simulink library "powerlib_extras"  (Simulink 6.0)
settings: Solver=ode45  SolverMode=SingleTasking  StartTime=0.0  StopTime=10.0  RelTol=1e-3
values from neighbouring files (symbols this model uses):
  Ts = get(handles.edit1,'string')    [powergui.m]
undefined symbols (not defined in the file or in its folder): Ac, Bc, Cc, Dc, Delay_discrete, dend, DiscIntNeverNeededParam, extra_sc, j, numd, test_alpha
libraries: powerlib2 x112, powerlib_extras x70, simulink_extras x25, simulink x12, powerlib_models x8
(part 2 of 9)

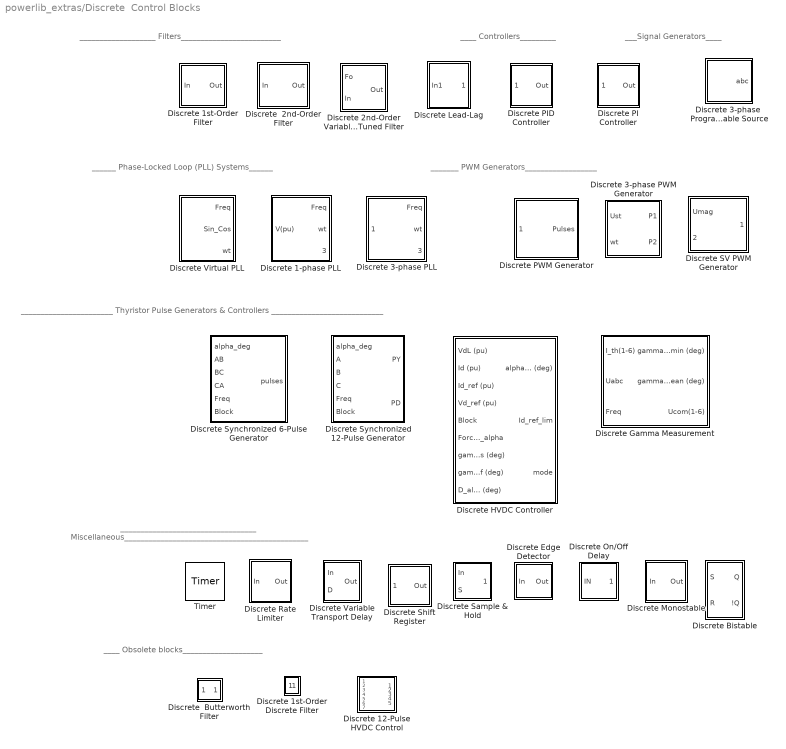
== system powerlib_extras/Discrete  Control Blocks ==
  note: ___________________ Filters_________________________
  note: ______ Phase-Locked Loop (PLL) Systems______
  note: _______________________ Thyristor Pulse Generators & Controllers ____________________________
  note: _______ PWM Generators__________________
  note: __________________________________ Miscellaneous______________________________________________
  note: ____ Controllers_________
  note: ___Signal Generators____
  note: ____ Obsolete blocks____________________
  Discrete 1-phase PLL : Subsystem  mask(Discrete 1-phase PLL){Fmin=45, Par_Init=[-45 60], ParK=[120 2800], Ts=50e-6}
      mask prompts: Fmin "Minimum frequency (Hz):"; Par_Init "Initial input:[ Phase(degrees)   Frequency(Hz) ]"; ParK "Regulator gains [ Kp  Ki ]"; Ts "Sample time:"
      mask help:
      | This Phase Locked Loop (PLL) system can be used  to synchronize on a variable frequency sinusoidal signal.
      |
      | Input 1: Normalized input signal V(pu)
      |
      | Output 1:  Measured frequency (Hz) = w/(2pi)
      | Output 2:  Ramp w.t  varying between  0 and 2*pi, synchronized on the zero-crossing (rising) of  the input signal
      | Output 3: Vector [sin(wt) cos(wt)]
      mask init:
      | Kp=ParK(1);
      | Ki=ParK(2);
      | Phase_Init=Par_Init(1);
      | Finit=Par_Init(2);
  Discrete 1st-Order Discrete Filter : Subsystem  mask(Discrete 1st-Order Filter){FilterType=Highpass, Tc=12e-3, Ts=50e-6, Initialize=off, Vac_Init=[0.8 -25 60], Vdc_Init=-0.4, PlotResponse=off, param1=[1 500 0.1]}
      mask prompts: FilterType "Filter Type:"; Tc "Time constant (s):"; Ts "Sample time:"; Initialize "Initialize filter states"; Vac_Init "AC initial input: [ Mag  Phase(degrees)  Freq(Hz) ]"; Vdc_Init "DC Initial input:"; PlotResponse "Plot filter response"; param1 "Frequency range(Hz) : [Start  End  Inc.]"
      mask init:
      | switch FilterType
      | case 1, % Lowpass
      |     X=[0 1 2 3 4];
      |     Y=[-2 -2 -3 -4 -4];
      |     numc=1;
      |     denc=[Tc 1];
      | case 2,   % Highpass
      |     X=[0 1 2 3 4];
      |     Y=[-4 -4 -3 -2 -2];
      |     numc=[1 0];
      |     denc=[1 1/Tc];
      | end
      | %
      | [Ac,Bc,Cc,Dc]=tf2ss(numc,denc);
      | %
      | %  Conversion to discrete transfer function
      | nstates = size(Ac,1);
      | invexp = inv(eye(nstates) - (Ts/2)*Ac);
      | Ad = invexp*(eye(nstates) + (Ts/2)*Ac);
      | Bd = invexp*Bc;
      | Cd = Cc*invexp*Ts;
      | Dd = Cc*invexp*Bc*(Ts/2) + Dc;
      | %
      | if Initialize==1  % Compute initial conditions on states
      |     u1=Vac_Init(1)*exp(j*Vac_Init(2)*pi/180);
      |     u2=Vdc_Init*exp(j*90*pi/180);
      |     u=u1+u2;
      |     u0=imag(u); % input at  t=0;
      |     I=eye(size(Ac));
      |     sI1=I*j*(2*pi*Vac_Init(3));
      |     sI2=I*j*0;
      |     x=inv(sI1-Ac)*Bc*u1 + inv(sI2-Ac)*Bc*u2;
      |     x0c=imag(x);
      |     x0d=(I-Ac*Ts/2)*x0c/Ts - Bc/2*u0;
      | else
      |     x0d=0;
      | end
      | 
      | %
      | if PlotResponse==1 % Plot frequency and step response
      | t=[0:Tc/1000:7*Tc];
      | f=param1(1):param1(3):param1(2);
      | w=2*pi*f;
      | switch FilterType
      | 	case 1, % Lowpass
      | 		Ystep=1 - exp(-t/Tc);
      | 		RepFreq=1./(1+Tc*j.*w);
      | 	case 2,   % Highpass
      | 		Ystep=exp(-t/Tc);
      | 		RepFreq=1./(1 + (1./(Tc*j.*w)));
      | end
      | %
      | Mag=abs(RepFreq);
      | Pha=angle(RepFreq)*180/pi;
      | %
      | figure(1)
      | subplot(2,1,1)
      | plot(f,Mag)
      | grid
      | title('Bode Diagram')
      | ylabel('Magnitude')
      | subplot(2,1,2)
      | plot(f,Pha)
      | ylabel('Phase (deg)')
      | xlabel('Frequency (Hz)')
      | grid
      | figure(2)
      | plot(t,Ystep)
      | grid
      | ylabel('Amplitude')
      | xlabel('Time (s)')
      | title('Step Response')
      | end
      mask StyleString: popup(Lowpass|Highpass),edit,edit,checkbox,edit,edit,checkbox,edit
      mask CallbackString: |||p4=get_param(gcb,'Initialize');if strcmp(p4,'on');visible={'on','on','on','on','on','on','on',get_param(gcb,'PlotResponse')};else;visible={'on','on','on','on','off','off','on',get_param(gcb,'PlotResponse')};end;set_param(gcb,'MaskVisibilities',visible)|||p7=get_param(gcb,'PlotResponse');if strcmp(p7,'on');visible={'on','on','on','on',get_param(gcb,'Initialize'),get_param(gcb,'Initialize'),'on','on'};else;visible={'on','on','on','on',get_param(gcb,'Initialize'),get_param(gcb,'Initialize'),'on','off'};end;set_param(gcb,'MaskVisibilities',visible)|
      mask Display: plot(X,Y);
  Discrete 1st-Order Filter : Subsystem  mask(Discrete 1st-Order Filter){FilterType=Highpass, Tc=12e-3, Ts=50e-6, Initialize=off, Vac_Init=[0.8 -25 60], Vdc_Init=-0.4, PlotResponse=off, param1=[1 500 0.1]}
      mask prompts: FilterType "Filter Type:"; Tc "Time constant (s):"; Ts "Sample time:"; Initialize "Initialize filter states"; Vac_Init "AC initial input: [ Mag  Phase(degrees)  Freq(Hz) ]"; Vdc_Init "DC Initial input:"; PlotResponse "Plot filter response"; param1 "Frequency range(Hz) : [Start  End  Inc.]"
      mask init: same as powerlib_extras/Discrete  Control Blocks/Discrete 1st-Order Discrete Filter
      mask StyleString: popup(Lowpass|Highpass),edit,edit,checkbox,edit,edit,checkbox,edit
      mask CallbackString: |||p4=get_param(gcb,'Initialize');if strcmp(p4,'on');visible={'on','on','on','on','on','on','on',get_param(gcb,'PlotResponse')};else;visible={'on','on','on','on','off','off','on',get_param(gcb,'PlotResponse')};end;set_param(gcb,'MaskVisibilities',visible)|||p7=get_param(gcb,'PlotResponse');if strcmp(p7,'on');visible={'on','on','on','on',get_param(gcb,'Initialize'),get_param(gcb,'Initialize'),'on','on'};else;visible={'on','on','on','on',get_param(gcb,'Initialize'),get_param(gcb,'Initialize'),'on','off'};end;set_param(gcb,'MaskVisibilities',visible)|
      mask Display: plot(X,Y);
  Discrete 2nd-Order Variable-Tuned Filter : Subsystem  mask(Discrete 2nd-Order Variable-Tuned Filter){FilterType=Bandpass, Fo=60, Zeta=1, Ts=50e-6, Initialize=off, Par_Init=[1.2 -30 30], Vdc=0}
      mask prompts: FilterType "Type of filter:"; Fo "Initial cut-off frequency Fo (Hz):"; Zeta "Damping factor Zeta ( Q = 1 / (2*Zeta) ):"; Ts "Sample Time: (s)"; Initialize "Initialize filter states"; Par_Init "AC initial input: [ Mag  Phase(degrees)  Freq(Hz) ]"; Vdc "DC initial input:"
      mask init:
      | switch FilterType
      | case 1, % Lowpass
      |        X=[0 1 2 3 4];
      |        Y=[-2 -2 -3 -4 -4];
      |  case 2,   % Highpass
      |        X=[0 1 2 3 4];
      |        Y=[-4 -4 -3 -2 -2];
      |     case 3,   % Bandpass
      |        X=[0 1 2 3 4 5 ];
      |        Y=[-3 -3 -2 -2 -3 -3];
      |     case 4,  %Bandstop (Notch)
      |        X=[0 1 2 3 4 5 ];
      |        Y=[-2 -2 -3 -3 -2 -2];
      |  end
      | Correction=3.549e6*Ts*Ts/60/60/60;
      | if Initialize==1
      | Vin=Par_Init(1)*(cos(Par_Init(2)*pi/180) + j*sin(Par_Init(2)*pi/180));
      | I=Vin/2/Zeta/(2*pi*Par_Init(3));
      | Wo=2*pi*Fo;
      | W=2*pi*Par_Init(3);
      | R=2*Zeta*Wo;
      | L=1;
      | C=1/(Wo*Wo);
      | I=Vin/(R + j*W*L -j/C/W);
      | Iinit=imag(I);
      | VL=imag(I * j*W*L);
      | VC=imag(I * -j/W/C)+ Vdc;
      | else
      | VC=0;
      | VL=0;
      | Iinit=0;
      | end
      mask StyleString: popup(Lowpass|Highpass|Bandpass|Bandstop (Notch)),edit,edit,edit,checkbox,edit,edit
      mask CallbackString: ||||p5=get_param(gcb,'Initialize');if strcmp(p5,'on');visible={'on','on','on','on','on','on','on'};else;visible={'on','on','on','on','on','off','off'};end;set_param(gcb,'MaskVisibilities',visible)||
      mask Display: plot(X,Y);
  Discrete 3-phase  Programmable Source : Subsystem  mask(Discrete 3-phase Programmable Source){Par_Vps=[1.0 -20  60], VariationEntity=Amplitude, VariationType=Step, VariationStep=-0.5, VariationRate=10, VariationMag=0.3, VariationFreq=2, Par_Timing_Variation=[0.1 1.2], SinglePhase=on, Yampli=[1 0.2 1.2 1.0], Xtime=[0 0.1 0.15 0.2], HarmonicGeneration=off, Par_HarmoA=[3 0.2 -25 0], Par_HarmoB=[2 0.15 35 2], Par_Timing_Harmo=[0.05  3], Ts=50e-6}
      mask prompts: Par_Vps "Positive-sequence: [ Amplitude  Phase(degrees)   Freq. (Hz) ]"; VariationEntity "Time variation of:"; VariationType "Type of variation:"; VariationStep "Step magnitude:"; VariationRate "Rate of change (value/s):"; VariationMag "Amplitude of the modulation:"; VariationFreq "Frequency of the modulation(Hz):"; Par_Timing_Variation "Variation timing (s) : [ Start   End ]"; SinglePhase "1-phase only"; Yampli "Amplitude values:"; Xtime "Time values:"; HarmonicGeneration "Harmonic generation:"; Par_HarmoA "A:  [ Order(n)   Amplitude  Phase(degrees)  Seq(0, 1 or 2) ]"; Par_HarmoB "B:  [ Order(n)   Amplitude  Phase(degrees)  Seq(0, 1 or 2) ]"; Par_Timing_Harmo "Harmonic timing (s) : [ Start   End ]"; Ts "Sample time:"
      mask help: Use this discrete block to generate a set of three-phase sinusoidal voltages or currents a, b and c. Time variation for the amplitude, phase and frequency of the fundamental can be pre-programmed. In addition, two harmonics can be surimposed on the fundamental.
      mask init:
      | Mag_Vps=Par_Vps(1);
      | Phase_Vps=Par_Vps(2);
      | Freq_Vps=Par_Vps(3);
      | 
      | Ton_Variation=Par_Timing_Variation(1);
      | Toff_Variation=Par_Timing_Variation(2);
      | n_HarmoA=Par_HarmoA(1);
      | Mag_HarmoA=Par_HarmoA(2);
      | Phase_HarmoA=Par_HarmoA(3);
      | Seq_HarmoA=Par_HarmoA(4);
      | if n_HarmoA==0
      |     Phase_HarmoA=90;
      |     Seq_HarmoA=0;
      | end
      | n_HarmoB=Par_HarmoB(1);
      | Mag_HarmoB=Par_HarmoB(2);
      | Phase_HarmoB=Par_HarmoB(3);
      | Seq_HarmoB=Par_HarmoB(4);
      | if n_HarmoB==0
      |     Phase_HarmoB=90;
      |     Seq_HarmoB=0;
      | end
      | Ton_Harmo=Par_Timing_Harmo(1);
      | Toff_Harmo=Par_Timing_Harmo(2);
      | 
      | if Xtime(1)~=0,
      | Xtime=[0 Xtime];
      | Yampli=[0 Yampli];
      | end
      | n=length(Xtime); vec_dt= [Xtime,0] - [0,Xtime] ; vec_dt=vec_dt(2:n);
      mask StyleString: edit,popup(None|Amplitude|Phase|Frequency),popup(Step|Ramp|Modulation|Table of time-amplitude pairs),edit,edit,edit,edit,edit,checkbox,edit,edit,checkbox,edit,edit,edit,edit
      mask CallbackString: |parametres=get_param(gcb,'MaskValues');p2=parametres{2};p3=parametres{3};p12=parametres{12};if strcmp(p3,'Step');param4='on';param5='off';param6='off';param7='off';param8='on';param9='off';param10='off';param11='off';elseif strcmp(p3,'Ramp');param4='off';param5='on';param6='off';param7='off';param8='on';param9='off';param10='off';param11='off';elseif strcmp(p3,'Modulation');param4='off';param5='off';param6='on';param7='on';param8='on';param9='off';param10='off';param11='off';else;param4='off';param5='off';param6='off';param7='off';param8='off';param9='on';param10='on';param11='on';end;if strcmp(p2,'None');param3='off';param4='off';param5='off';param6='off';param7='off';param8='off';param9='off';param10='off';param11='off';else;param3='on';end;if strcmp(p12,'on');param13='on';param14='on';param15='on';else;param13='off';param14='off';param15='off';end;visible={'on','on',param3,param4,param5,param6,param7,param8,param9,param10,param11,'on',param13,param14,param15,'on'};set_param(gcb,'MaskVisibilities',visible)|parametres=get_param(gcb,'MaskValues');p2=parametres{2};p3=parametres{3};p12=parametres{12};if strcmp(p3,'Step');param4='on';param5='off';param6='off';param7='off';param8='on';param9='off';param10='off';param11='off';elseif strcmp(p3,'Ramp');param4='off';param5='on';param6='off';param7='off';param8='on';param9='off';param10='off';param11='off';elseif strcmp(p3,'Modulation');param4='off';param5='off';param6='on';param7='on';param8='on';param9='off';param10='off';param11='off';else;param4='off';param5='off';param6='off';param7='off';param8='off';param9='on';param10='on';param11='on';end;if strcmp(p2,'None');param3='off';param4='off';param5='off';param6='off';param7='off';param8='off';param9='off';param10='off';param11='off';else;param3='on';end;if strcmp(p12,'on');param13='on';param14='on';param15='on';else;param13='off';param14='off';param15='off';end;visible={'on','on',param3,param4,param5,param6,param7,param8,param9,param10,param11,'on',param13,param14,param15,'on'};set_param(gcb,'MaskVisibilities',visible)|||||||||parametres=get_param(gcb,'MaskValues');p2=parametres{2};p3=parametres{3};p12=parametres{12};if strcmp(p3,'Step');param4='on';param5='off';param6='off';param7='off';param8='on';param9='off';param10='off';param11='off';elseif strcmp(p3,'Ramp');param4='off';param5='on';param6='off';param7='off';param8='on';param9='off';param10='off';param11='off';elseif strcmp(p3,'Modulation');param4='off';param5='off';param6='on';param7='on';param8='on';param9='off';param10='off';param11='off';else;param4='off';param5='off';param6='off';param7='off';param8='off';param9='on';param10='on';param11='on';end;if strcmp(p2,'None');param3='off';param4='off';param5='off';param6='off';param7='off';param8='off';param9='off';param10='off';param11='off';else;param3='on';end;if strcmp(p12,'on');param13='on';param14='on';param15='on';else;param13='off';param14='off';param15='off';end;visible={'on','on',param3,param4,param5,param6,param7,param8,param9,param10,param11,'on',param13,param14,param15,'on'};set_param(gcb,'MaskVisibilities',visible)||||
  Discrete 3-phase PLL : Subsystem  mask(Discrete 3-phase PLL){Fmin=45, Par_Init=[-45 60], ParK=[60 1400], Ts=50e-6}
      mask prompts: Fmin "Minimum frequency (Hz):"; Par_Init "Initial inputs:[ Phase(degrees)   Frequency(Hz) ]"; ParK "Regulator gains [ Kp  Ki ]"; Ts "Sample time:"
      mask help:
      | This Phase Locked Loop (PLL) system can be used  to synchronize on a set of variable frequency, three-phase sinusoidal signals.
      |
      | Input 1: Vector containing the normalized
      |              three-phase signals [Va Vb Vc]
      | Output 1:  Measured frequency (Hz) = w/(2pi)
      | Output 2:  Ramp w.t   varying between  0 and 2*pi,
      | synchronized on zero crossings of the fundamental (positive-sequence) of phase A.
      | Output 3: Vector [sin(wt) cos(wt)]
      mask init:
      | Kp=ParK(1);
      | Ki=ParK(2);
      | Phase_Init=Par_Init(1);
      | Finit=Par_Init(2);
  Discrete Bistable : Subsystem  AncestorBlock=my_linear/BETA/Flip flop [R]  mask(Discrete Bistable Flip-Flop (Priority to Set or Reset)){priority=Set, ic=0, Ts=50e-6}
      mask prompts: priority "Priority to input:"; ic "Initial Q output (0/1):"; Ts "Sample time:"
      mask help:
      | SR Flip-Flop block, with priority given either  to the Set  (S) or Reset  (R) input.
      |
      | Priority to Set: If inputs S (set) and R (reset) are TRUE (1) simultaneously, the output Q is set to TRUE (1).
      |
      | Priority to Reset: If inputs S (set) and R (reset) are TRUE (1) simultaneously, the output Q is reset to FALSE (0).
      |
      | The  Q! output  is the complement of the Q output.
      | The initial value of the Q output  is specified by the parameter "Initial Q output".
      mask init:
      | if (priority==1)   % RESET
      |  str1 = '[R]';
      |  str2 = 'S';
      | else
      | str1= 'R';
      | str2 = '[S]';
      | end
      mask StyleString: popup(Reset|Set),edit,edit
      mask Display:
      | plot(0,0,100,100);
      | text(5,25,str1);
      | text(5,75,str2);
      | text(72,25,'!Q');
      | text(78,75,'Q');
  Discrete Edge Detector : Subsystem  mask(Discrete Edge Detector){model=Rising, ic=0, Ts=50e-6}
      mask prompts: model "Edge:"; ic "Input at t = -Ts:"; Ts "Sample time Ts:"
      mask help:
      | This block compares its present input to its previous input.
      |
      | If the input  is a logic signal (TRUE (1) or FALSE (0), the output is a one-step boolean signal TRUE  when  the specified edge (Rising, Falling or Either)  is detected.
      |
      | This block can also be used to detect the slope polarity of a continuous signal. For example, if the specified edge is  "Rising", the output is TRUE as long as the slope of the input signal is positive.
      |
      | The input value at time step preceeding t=0 is specified by the parameter "Input at t=-Ts"
      mask init: same as powerlib_extras/Control  Blocks/Edge Detector
      mask StyleString: popup(Rising|Falling|Either),edit,edit
      mask Display: plot(0,0,100,100, X1,Y1,X2,Y2,X3,Y3,X4,Y4);
  Discrete Lead-Lag : Subsystem  mask(Discrete Lead-Lag Controller){T1=5e-3, T2=20e-3, V_Init=0, Ts=50e-6}
      mask prompts: T1 "Time constant T1 (s):"; T2 "Time constant T2 (s):"; V_Init "Initial input and output:"; Ts "Sample time (s):"
      mask help:
      | This block implements a discrete lead-lag controller:
      |
      |          1+T1s
      | H(s)= ------
      |          1+T2s
      |
      | States are initialized according to initial input anf output value so that simulation starts in steady state.
      mask init:
      | numc=[T1 1];
      | denc=[T2 1];
      | [Ac,Bc,Cc,Dc]=tf2ss(numc,denc);
      | 
      | %  Conversion to discrete transfer function
      | nstates = size(Ac,1);
      | invexp = inv(eye(nstates) - (Ts/2)*Ac);
      | Ad = invexp*(eye(nstates) + (Ts/2)*Ac);
      | Bd = invexp*Bc;
      | Cd = Cc*invexp*Ts;
      | Dd = Cc*invexp*Bc*(Ts/2) + Dc;
      | %
      | % Compute Initial states
      | I=eye(size(Ac));
      | x0c=inv(-Ac)*Bc*V_Init;
      | x0d=(I-Ac*Ts/2)*x0c/Ts - Bc/2*V_Init;
      | 
      | if T1==0 & T2==0, Dd=1; end
      mask Display: disp('1+T1s\n---\n1+T2s')
  Discrete Monostable : Subsystem  mask(Discrete Monostable Flip-Flop){EdgeDetect=Rising, t_mono=0.015, ic=0, Ts=50e-6}
      mask prompts: EdgeDetect "Edge detection"; t_mono "Pulse duration (s):"; ic "Input at t = -Ts:"; Ts "Sample time Ts:"
      mask help:
      | After being triggered  by the specified edge (Rising, Falling or Either), this block outputs a pulse (TRUE signal) for the time specified by parameter "Pulse duration".
      | If the specified edge is detected while the output is TRUE, the monostable is not retriggered
      |
      | The input value (0/1) at time step preceeding t = 0 is specified by the parameter "input at t = -Ts.
      mask init: same as powerlib_extras/Control  Blocks/Monostable
      mask StyleString: popup(Rising|Falling|Either),edit,edit,edit
      mask Display:
      | plot(0,0,100,100,[100 75 75 25 25 0],[25 25 50 50 25 25]-0,X1,Y1,X2,Y2,X3,Y3,X4,Y4);
      | text(45,37,'T');
      | text(15,15,str);
  Discrete On/Off Delay : Subsystem  AncestorBlock=extra_sc/Delay_discrete  mask(Discrete On/Off Delay ){type_delay=On delay, delay=0.01, ic=0, Ts=50e-6}
      mask prompts: type_delay "Type:"; delay "Time delay:"; ic "Input at t = -Ts (0/1):"; Ts "Sample time Ts:"
      mask help:
      | Apply a delay on the input signal when the input changes to TRUE (1) or FALSE (0).
      |
      | On delay: When the input becomes TRUE, the output becomes TRUE after the specified time delay as long as the input is still TRUE. If the input becomes FALSE before the time delay has expired , the output stays FALSE.
      |
      | Off delay: When the input becomes FALSE, the output becomes FALSE after the specified time delay as long as the input is still FALSE. If the input becomes TRUE before the time delay has expired , the output stays TRUE.
      |
      | The input value (0/1) at time step preceeding t=0 is specified by the parameter "input at t = -Ts".
      mask init:
      | str=sprintf('%g %c',delay,'s');
      mask StyleString: popup(On delay|Off delay),edit,edit,edit
      mask Display:
      | plot(0,0,100,100,[10,10,10,90,90,90],[60,40,50,50,40,60]);
      | text(25+(type_delay-1)*50,80,'t');
      | text(15,20,str);
  Discrete PI Controller : Subsystem  mask(Discrete PI Controller){Kp=0.1, Ki=1, Par_Limits=[1e6 -1e6], Init=0, Ts=50e-6}
      mask prompts: Kp "Proportional gain (Kp):"; Ki "Integral gain (Ki):"; Par_Limits "Output limits: [ Upper   Lower ]"; Init "Output initial value:"; Ts "Sample time:"
      mask help: This block implements a discrete PI controller.
      mask init:
      | UpperLimit=Par_Limits(1);
      | LowerLimit=Par_Limits(2);
      mask Display: disp('PI');
  Discrete PID Controller : Subsystem  mask(Discrete PID Controller){Kp=0.1, Ki=1, Kd=0, TcD=0.5e-3, Par_Limits=[1e6 -1e6], Init=0, Ts=50e-6}
      mask prompts: Kp "Proportional gain (Kp):"; Ki "Integral gain (Ki):"; Kd "Derivative gain (Kd):"; TcD "Time constant for derivative (s):"; Par_Limits "Output limits: [ Upper   Lower ]"; Init "Output initial value:"; Ts "Sample time:"
      mask help: This block implements a discrete PID controller.
      mask init:
      | UpperLimit=Par_Limits(1);
      | LowerLimit=Par_Limits(2);
      mask Display: disp('PID');
  Discrete PWM Generator : Subsystem  mask(Discrete PWM Generator){GeneratorMode=2-arm  bridge (4 pulses), Fc=1080, Ts=5e-6, Internal=off, mIndex=0.4, Freq=60, Phase=0}
      mask prompts: GeneratorMode "Generator Mode"; Fc "Carrier frequency (Hz):"; Ts "Sample time:"; Internal "Internal generation of modulating signal(s)"; mIndex "Modulation index  (0<m<1) :"; Freq "Frequency of output voltage (Hz)"; Phase "Phase of output voltage (degrees)"
      mask help:
      | This discrete block generates pulses for carrier-based PWM (Pulse Width Modulation), self-commutated IGBTs,GTOs or FETs bridges.
      |
      | Depending on the number of bridge arms selected in the "Generator Mode" parameter, the block can be used either for single-phase or three-phase PWM control.
      |
      | Press Help for details on input(s) and outputs.
      |
      | See psb1phPWM and psb3phPWM demos respectively  for application examples of single-phase and three-phase inverters using this block.
      mask init:
      | powericon('psbcbtransfo',gcb,'Discrete PWM Generator')
      | if Freq==0
      |     Phase=90;
      | end
      | switch GeneratorMode
      | case 1,
      |     Internal_Phase=0;
      |    Signal_PortWidth=1;
      |    Select1_Elements=[1 2];
      |    Select1_PortWidth=2;
      |    Select3_Elements=[1 2];
      |    Select3_PortWidth=4;
      | case 2,
      |     Internal_Phase=0;
      |     Signal_PortWidth=1;
      |     Select1_Elements=[1 2];
      |     Select1_PortWidth=2;
      |     Select3_Elements=[1 2 3 4];
      |     Select3_PortWidth=4;
      | case 3,
      |     Internal_Phase=[0 -2*pi/3 2*pi/3];
      |     Signal_PortWidth=3;
      |     Select1_Elements=[1 4 2 5 3 6];
      |     Select1_PortWidth=6;
      |    Select3_Elements=[1 2 3 4 5 6];
      |    Select3_PortWidth=12;
      | case 4,
      |     Internal_Phase=[0 -2*pi/3 2*pi/3];
      |     Signal_PortWidth=3;
      |     Select1_Elements=[1 4 2 5 3 6];
      |     Select1_PortWidth=6;
      |    Select3_Elements=[1 2 3 4 5 6 7 8 9 10 11 12];
      |    Select3_PortWidth=12;
      | end
      mask Help:
      | The output pulses are a vector (with values=0 or 1). Depending on the selected "Generator Mode", the output vector contains:
      | For a 1-arm  bridge: Two pulses. Pulse 1 is for the upper switch and pulse 2 is for the lower switch.
      | For a 2-arm  bridge: Four pulses. Pulses 1 and 3 are respectively for the upper switches of the first and second arm. Pulses 2 and 4 are for the lower switches.
      | For a 3-arm  bridge: Six pulses. Pulses 1,3 and 5 are respectively for the upper switches of the first,second and third arm. Pulses 2,4 and 6 are for the lower switches.
      | For double 3-arm bridges: Twelve pulses.The first six pulses (pulses 1 to 6) must be sent to the first 3-arm bridge and the last six (pulses 7 to 12) to the second 3-arm bridge.
      | 
      | By selecting "Internal generation" you can can control the modulation index m, frequency and phase of the output voltage  from the internal parameters (m, Freq and Phase). Otherwise, external signals are used for pulse generation. The width of the input vector must be 1 for single phase bridges ( 1-arm or 2-arm)  and 3 for 3-phase bridges  (single or double bridge).
      mask StyleString: popup(1-arm  bridge (2 pulses)|2-arm  bridge (4 pulses)|3-arm  bridge (6 pulses)|Double 3-arm  bridges (12 pulses)),edit,edit,checkbox,edit,edit,edit
      mask CallbackString: |||powericon('psbcbtransfo',gcb,'Discrete PWM Generator',[])|||
  Discrete Rate Limiter : Subsystem  mask{R=2000, F=-2000, Vinit=0, Ts=50e-6}
      mask prompts: R "Rising slew rate:"; F "Falling slew rate:"; Vinit "Initial input:"; Ts "Sample time:"
      mask help: DISCRETE BLOCK : Limit rising and falling rates of signal
      mask init:
      | UpperLimit=R*Ts;
      | LowerLimit=F*Ts;
      mask Display: disp('Discrete\nRate\nLimiter')
  Discrete Sample & Hold : Subsystem  mask(Discrete Sample & Hold ){ic=0, Ts=50e-6}
      mask prompts: ic "Initial condition:"; Ts "Sample time:"
      mask help: The output follows input 1 (In) as long as input 2 (S) is TRUE (1) . The output is held when input 2 becomes FALSE (0). The output initial value is specified by the parameter "Initial condition".
      mask Display: disp('S/H')
  Discrete Shift Register : Subsystem  mask(Discrete Shift Register){NSamples=32, InitialValue=0, Ts=50e-6}
      mask prompts: NSamples "Number of samples N :"; InitialValue "Initial inputs:"; Ts "Sample time Ts:"
      mask help:
      | This block implements a discrete shift register (Serial input/ Parallel output). The block accepts a vectorized input of Nsig signals.
      |
      | The block output is a vector (dimension N*Nsig) containing the last N samples of the Nsig input signals in the following order
      | [u1(k), u1(k-1), ..., u1(k-(N-1)),  u2(k), u2(k-1), ...]
      |
      | The (N-1) samples preceding time zero are set to the  value specified in the "Initial inputs" parameter.
  Discrete Virtual PLL : Subsystem  mask(Discrete Virtual PLL){Freq=60, Phase=30, Ts=50e-6}
      mask prompts: Freq "Frequency (Hz):"; Phase "Phase (degrees):"; Ts "Sample time:"
      mask help:
      | This virtual PLL has no input signal. The block simulates the outputs of an actual PLL by  using the parameters specified in the mask.
      |
      | Output 1: Frequency (Hz)
      | Output 2: Vectorized output  [sin(wt)  cos(wt)]
      | Output 3: wt in rad/s (varying from 0 to 2*pi)
  Discrete  2nd-Order Filter : Subsystem  mask(Discrete 2nd-Order Filter){FilterType=Lowpass, Fo=200, Zeta=0.707, Ts=50e-6, Initialize=off, Vac_Init=[0.8 -25 60], Vdc_Init=-0.4, PlotResponse=off, param1=[1 500 1]}
      mask prompts: FilterType "Filter Type:"; Fo "Cut-off frequency (Hz):"; Zeta "Damping factor Zeta ( Q = 1 / (2*Zeta) ):"; Ts "Sample time:"; Initialize "Initialize filter states"; Vac_Init "AC initial input: [ Mag  Phase(degrees)  Freq(Hz) ]"; Vdc_Init "DC Initial input:"; PlotResponse "Plot filter response"; param1 "Frequency range(Hz) : [Start  End  Inc.]"
      mask init:
      | str=sprintf(' Fo=%iHz\n\n',Fo);
      | Wo=2*pi*Fo;
      | switch FilterType
      | case 1, % Lowpass
      |        X=[0 1 2 3 4];
      |        Y=[-2 -2 -3 -4 -4];
      |        n2=0;n1=0;n0=Wo*Wo;
      |        d2=1;d1=2*Zeta*Wo;d0=Wo*Wo;
      | 	   Ystep=1;
      |  case 2,   % Highpass
      |        X=[0 1 2 3 4];
      |        Y=[-4 -4 -3 -2 -2];
      |        n2=1;n1=0;n0=0;
      |        d2=1;d1=2*Zeta*Wo;d0=Wo*Wo;
      | 	   Ystep=2;
      |     case 3,   % Bandpass
      |        X=[0 1 2 3 4 5 ];
      |        Y=[-3 -3 -2 -2 -3 -3];
      |        n2=0;n1=2*Zeta*Wo;n0=0;
      |        d2=1;d1=2*Zeta*Wo;d0=Wo*Wo;
      | 	   Ystep=3;
      |     case 4,  %Bandstop (Notch)
      |        X=[0 1 2 3 4 5 ];
      |        Y=[-2 -2 -3 -3 -2 -2];
      |        n2=1;n1=0;n0=Wo*Wo;
      |        d2=1;d1=2*Zeta*Wo;d0=Wo*Wo;
      | 	   Ystep=4;
      |     end
      | %
      | numc=[n2 n1 n0];
      | denc=[d2 d1 d0];
      | [Ac,Bc,Cc,Dc]=tf2ss(numc,denc);
      | %
      | %  Conversion to discrete transfer function
      | nstates = size(Ac,1);
      | invexp = inv(eye(nstates) - (Ts/2)*Ac);
      | Ad = invexp*(eye(nstates) + (Ts/2)*Ac);
      | Bd = invexp*Bc;
      | Cd = Cc*invexp*Ts;
      | Dd = Cc*invexp*Bc*(Ts/2) + Dc;
      | %
      | if Initialize==1  % Compute initial conditions on states
      | u1=Vac_Init(1)*exp(j*Vac_Init(2)*pi/180);
      | u2=Vdc_Init*exp(j*90*pi/180);
      | u=u1+u2;
      | u0=imag(u); % input at  t=0;
      | I=eye(size(Ac));
      | sI1=I*j*(2*pi*Vac_Init(3));
      | sI2=I*j*0;
      | x=inv(sI1-Ac)*Bc*u1 + inv(sI2-Ac)*Bc*u2;
      | x0c=imag(x);
      | x0d=(I-Ac*Ts/2)*x0c/Ts - Bc/2*u0;
      | else
      | x0d=0;
      | end
      | %
      | if PlotResponse==1 % Plot frequency and step response
      | if Zeta==1
      | 	z=1+1e-12;
      | else
      | 	z=Zeta;
      | end
      | wn=Wo;
      | t=[0:1/(z*wn)/1000:7/(z*wn)];
      | f=param1(1):param1(3):param1(2);
      | w=2*pi*f;
      | switch FilterType
      | 	case 1, % Lowpass
      | 		Ystep=wn^2*(1/wn^2+1/(4*z^2*wn^2-4*wn^2)^(1/2)*(1/(-z*wn+1/2*(4*z^2*wn^2-4*wn^2)^(1/2))*exp((-z*wn+1/2*(4*z^2*wn^2-4*wn^2)^(1/2))*t)-1/(-z*wn-1/2*(4*z^2*wn^2-4*wn^2)^(1/2))*exp((-z*wn-1/2*(4*z^2*wn^2-4*wn^2)^(1/2))*t)));
      | 		numFreq=wn^2;
      | 	case 2,   % Highpass
      | 		Ystep=-exp(-z*wn*t)/(z-1)/(z+1).*cos((-wn^2*(z-1)*(z+1))^(1/2)*t)+exp(-z*wn*t)/(z-1)/(z+1)*z^2.*cos((-wn^2*(z-1)*(z+1))^(1/2)*t)+z/wn*exp(-z*wn*t)/(z-1)/(z+1)*(wn^2-z^2*wn^2)^(1/2).*sin((-wn^2*(z-1)*(z+1))^(1/2)*t);
      | 		numFreq=-w.^2;
      | 	case 3,   % Bandpass
      | 		Ystep=2*z*wn/(4*z^2*wn^2-4*wn^2)^(1/2)*(exp((-z*wn+1/2*(4*z^2*wn^2-4*wn^2)^(1/2))*t)-exp((-z*wn-1/2*(4*z^2*wn^2-4*wn^2)^(1/2))*t));
      | 		numFreq=2*Zeta*wn.*w*j;
      | 	case 4,  %Bandstop (Notch)
      | 		Ystep=1+2*z/wn*exp(-z*wn*t)/(z-1)/(z+1)*(wn^2-z^2*wn^2)^(1/2).*sin((-wn^2*(z-1)*(z+1))^(1/2)*t);	
      | 		numFreq=wn^2-w.^2;
      | end
      | %
      | denFreq=(wn^2-w.^2) + 2*Zeta*wn*j.*w;
      | RepFreq=numFreq./denFreq;
      | Mag=abs(RepFreq);
      | Pha=angle(RepFreq)*180/pi;
      | %
      | figure(1)
      | subplot(2,1,1)
      | plot(f,Mag)
      | grid
      | title('Bode Diagram')
      | ylabel('Magnitude')
      | subplot(2,1,2)
      | plot(f,Pha)
      | ylabel('Phase (deg)')
      | xlabel('Frequency (Hz)')
      | grid
      | figure(2)
      | plot(t,real(Ystep))
      | grid
      | ylabel('Amplitude')
      | xlabel('Time (s)')
      | title('Step Response')
      | end
      mask StyleString: popup(Lowpass|Highpass|Bandpass|Bandstop (Notch)),edit,edit,edit,checkbox,edit,edit,checkbox,edit
      mask CallbackString: ||||p5=get_param(gcb,'Initialize');if strcmp(p5,'on');visible={'on','on','on','on','on','on','on','on',get_param(gcb,'PlotResponse')};else;visible={'on','on','on','on','on','off','off','on',get_param(gcb,'PlotResponse')};end;set_param(gcb,'MaskVisibilities',visible)|||p8=get_param(gcb,'PlotResponse');if strcmp(p8,'on');visible={'on','on','on','on','on',get_param(gcb,'Initialize'),get_param(gcb,'Initialize'),'on','on'};else;visible={'on','on','on','on','on',get_param(gcb,'Initialize'),get_param(gcb,'Initialize'),'on','off'};end;set_param(gcb,'MaskVisibilities',visible)|
      mask Display:
      | plot(X,Y);
      | disp(str);
  "Discrete  Butterworth Filter " : Subsystem  mask(Discrete Butterworth Filter){FilterType=Lowpass, N=2, Fo=80, Bo=80, Ts=50e-6, Initialize=on, Vac_Init=[1.2 60 60], Vdc_Init=-0.6, PlotResponse=off, param1=[1 500 0.1]}
      mask prompts: FilterType "Filter Type:"; N "Order(N) (Order=2*N for bandpass and bandstop)"; Fo "Cut-off frequency (Hz):"; Bo "Bandwith for bandpass and bandstop (Hz):"; Ts "Sample time:"; Initialize "Initialize filter states"; Vac_Init "AC initial input: [ Mag  Phase(degrees)  Freq(Hz) ]"; Vdc_Init "DC Initial input:"; PlotResponse "Plot filter response"; param1 "Frequency range(Hz) : [Start  End  Inc.]"
      mask init:
      | Wo=2*pi*Fo;
      | str=sprintf(' Fo= %iHz\nN= %i\n\n',Fo,N);
      | switch FilterType
      | case 1 % Lowpass
      |        X=[0 1 2 3 4];
      |        Y=[-2 -2 -3 -4 -4];
      |         [B,A]=butter(N,2*Fo*pi,'s');
      |  case 2 % Highpass
      |        X=[0 1 2 3 4];
      |        Y=[-4 -4 -3 -2 -2];
      |        [B,A]=butter(N,2*Fo*pi,'high','s');
      |     case 3 % Bandpass
      |        X=[0 1 2 3 4 5 ];
      |        Y=[-3 -3 -2 -2 -3 -3];
      |       [B,A]=butter(N,[2*pi*(Fo-Bo/2)  2*pi*(Fo+Bo/2)],'s');
      |     case 4  %Bandstop (Notch)
      |        X=[0 1 2 3 4 5 ];
      |        Y=[-2 -2 -3 -3 -2 -2];
      |       [B,A]=butter(N,[2*pi*(Fo-Bo/2)  2*pi*(Fo+Bo/2)],'stop','s');
      | end
      | [Ac,Bc,Cc,Dc]=tf2ss(B,A);
      | %  Conversion to discrete transfer function
      | nstates = size(Ac,1);
      | invexp = inv(eye(nstates) - (Ts/2)*Ac);
      | Ad = invexp*(eye(nstates) + (Ts/2)*Ac);
      | Bd = invexp*Bc;
      | Cd = Cc*invexp*Ts;
      | Dd = Cc*invexp*Bc*(Ts/2) + Dc;
      | %
      | %
      | if Initialize==1  % Compute initial conditions on states
      | u1=Vac_Init(1)*exp(j*Vac_Init(2)*pi/180);
      | u2=Vdc_Init*exp(j*90*pi/180);
      | u=u1+u2;
      | u0=imag(u); % input at  t=0;
      | I=eye(size(Ac));
      | sI1=I*j*(2*pi*Vac_Init(3));
      | sI2=I*j*0;
      | x=inv(sI1-Ac)*Bc*u1 + inv(sI2-Ac)*Bc*u2;
      | x0c=imag(x);
      | x0d=(I-Ac*Ts/2)*x0c/Ts - Bc/2*u0;
      | else
      | x0d=0;
      | end
      | %
      | if PlotResponse==1 % Plot frequency and step response
      | figure(1)
      | sys=ss(Ad,Bd,Cd,Dd,Ts);
      | f=param1(1):param1(3):param1(2);
      | w=2*pi*f;
      | [mag phase]=bode(sys,w);
      | subplot(2,1,1)
      | plot(f,squeeze(mag))
      | title('Magnitude')
      | grid
      | subplot(2,1,2)
      | plot(f,squeeze(phase))
      | title('Phase (degrees)')
      | xlabel('Hz')
      | grid
      | figure(2)
      | step(sys)
      | end
      mask StyleString: popup(Lowpass|Highpass|Bandpass|Bandstop (Notch)),edit,edit,edit,edit,checkbox,edit,edit,checkbox,edit
      mask CallbackString: |||||p6=get_param(gcb,'Initialize');if strcmp(p6,'on');visible={'on','on','on','on','on','on','on','on','on',get_param(gcb,'PlotResponse')};else;visible={'on','on','on','on','on','on','off','off','on',get_param(gcb,'PlotResponse')};end;set_param(gcb,'MaskVisibilities',visible)|||p9=get_param(gcb,'PlotResponse');if strcmp(p9,'on');visible={'on','on','on','on','on','on',get_param(gcb,'Initialize'),get_param(gcb,'Initialize'),'on','on'};else;visible={'on','on','on','on','on','on',get_param(gcb,'Initialize'),get_param(gcb,'Initialize'),'on','off'};end;set_param(gcb,'MaskVisibilities',visible)|
      mask Display:
      | plot(X,Y);
      | disp(str);
  "Discrete 12-Pulse HVDC Control " : Subsystem  mask(Discrete 12-pulse HVDC Control){Mode=Rectifier, f0Pw=[60 101.5], XPILimR=[165, 5], XLinR=[60, 20], XPILimI=[165, 92], XLinI=[160,  120], Xmarg=[0.1,  0.05], XKPI_I=[46, 4600, 90], XKPI_V=[36, 2256,  90], T1_I=0.3e-3, XT_V=[10e-3 , 0.1e-3], BP=45, Xvdcol=[0.6, 0.18, 0.30, 0.1, 0.080], alpha_const=off, alpha_fix=165, pas=50e-6}
      mask prompts: Mode "Control Mode :"; f0Pw "{Synchronisation} : [ BaseFrequency (Hz)  PulseWidth (deg) :"; XPILimR "{Rectifier} : [alpha max (deg), alpha min (deg) ]"; XLinR "{Rectifier} Kp Lin. Angle Limits: [Max  (deg), Min  (deg) ]"; XPILimI "{Inverter}  [alpha max (deg), alpha min (deg) ]"; XLinI "{Inverter} Kp Lin.  Angle Limits: [Max  (deg), Min  (deg) ]"; Xmarg "{Inverter} Current & Voltage Margin: [Id marg (pu) , Vd marg (pu) ]"; XKPI_I "{Current Regulator}   [Kp (pu) , Ki (pu/deg/s), AlphaInit (deg) ]"; XKPI_V "{Voltage Regulator}   [Kp (pu) , Ki (pu/deg/s),  AlphaInit(deg) ]"; T1_I "{Id Meas. Filter} H(s)=1/(1+T1s) : T1 (s)"; XT_V "{Vd Meas. Filter} H(s)=1/(1+T1s)(1+T2s) :  [T1 (s), T2 (s) ]"; BP "{Synchro. Band-Pass Filter}  Bandwidth  (Hz) :"; Xvdcol "{VDCOL}  [ VdThresh. (pu) , VdMin (pu), IdMin (pu), IdMinAbs (pu), Tup (s) ]"; alpha_const "Constant alpha mode"; alpha_fix "Alpha value (deg) (Constant alpha mode or Forced alpha):"; pas "Sample Time (s):"
      mask help:
      | This block generates the pulses required by a 12-pulse HVDC rectifier or inverter.
      | See the 'HVDC Transmission System' case study of the User's Manual
      | for description of the block functionality.
      | Press help for description of inputs and outputs.
      mask init:
      | f0=f0Pw(1); Pw=f0Pw(2);
      | Id_marg = Xmarg(1); Vd_marg = Xmarg(2);
      | alpha_max_rec = XPILimR(1); alpha_min_rec = XPILimR(2);
      | max_lin_rec = XLinR(1); min_lin_rec = XLinR(2);
      | alpha_max_inv = XPILimI(1); alpha_min_inv = XPILimI(2);
      | max_lin_inv = XLinI(1); min_lin_inv = XLinI(2);
      | Kp_I = XKPI_I(1); Ki_I = XKPI_I(2); ICi_I = XKPI_I(3);
      | Kp_V = XKPI_V(1); Ki_V = XKPI_V(2); ICi_V = XKPI_V(3);
      | T1_V = XT_V(1); T2_V = XT_V(2);
      | 
      | 
      | Vd_seuil = Xvdcol(1); Vd_min=Xvdcol(2);Id_min=Xvdcol(3);Id_min_abs=Xvdcol(4);Tup=Xvdcol(5);
      | if strcmp(alpha_const,'on'), test_alpha=1; else, test_alpha=0; end
      mask Help:
      | INPUTS:
      | Vabc  : 3 phase-to-ground voltages (pu)  on the primary winding of the YgYD              converter transformer
      | VdL     : DC line voltage (pu)
      | Id        : DC line current (pu)
      | Id_ref  : DC reference current (pu)
      | Vd_ref : DC line reference voltage (pu).  (Set Vd_ref  to a high value  (i.e. 2 pu) to disabble the voltage control in rectifier mode)
      | Block  : Logical signal  (0-1). (The converter is blocked when the value is 1)
      | ForcedDelay : Logical signal (0-1) used for protection . (When the value is 1  the alpha angle is forced  to the Constant alpha value.)
      | 
      | OUTPUTS:
      |  PulsesY :  6 pulses to be sent to the half converter connected to the Wye winding.
      |  PulsesD :  6 pulses to be sent to the half converter connected to the Delta winding.
      | alpha : firing angle of thyristors (degrees).
      | Id_ref_lim :Effective current order (limited Id_ref) applied to the current controler (pu).
      | Mode:  Number (0 to 5) indicating the actual control mode as follow: 0- Blocked pulses; 1- Current control;  2- Voltage control;
      | 3- Alpha minimum limitation; 4- Alpha maximum limitation; 5- Forced or constant alpha.
      mask StyleString: popup(Rectifier|Inverter),edit,edit,edit,edit,edit,edit,edit,edit,edit,edit,edit,edit,checkbox,edit,edit
      mask CallbackString: mode=get_param(gcb,'Mode');cb=get_param(gcb,'MaskVisibilities');if strcmp(mode,'Rectifier'),cb{3}='on';cb{4}='on';cb{5}='off';cb{6}='off';cb{7}='off';set_param(gcb,'MaskVisibilities',cb);else,cb{5}='on';cb{6}='on';cb{7}='on';cb{3}='off';cb{4}='off';set_param(gcb,'MaskVisibilities',cb);end|||||||||||||||
      mask Display: disp(',')
  Discrete 3-phase PWM Generator : Subsystem  mask(Discrete 3-phase PWM Generator (2- or 3-level)){ModulatorType=2-level, ModulatorMode=Synchronized, nF=18, Fc=18*60, ModulatingSignals=off, m=0.2, Freq=60, Phase=0, Ts=5e-6}
      mask prompts: ModulatorType "Type"; ModulatorMode "Mode of operation"; nF "Switching ratio: chopping frequency / output frequency"; Fc "Carrier frequency (Hz):"; ModulatingSignals "Internal generation of modulating signal(s)"; m "Modulation Index:"; Freq "Output voltage frequency (Hz):"; Phase "Output voltage phase (degrees):"; Ts "Sample time:"
      mask help:
      | The Discrete 3-phase PWM Generator block generates pulses for carrier-based Pulse Width Modulation (PWM) converters.
      | The block can be used to fire the forced-commuted devices (FETs, GTOs, or IGBTs) of 2-level or 3-level converters using a single  bridge or two bridges connected in twin configuration.
      | Vectorized outputs P1 and P2 contain  either 6 pulses (2-level) or 12 pulses (3-level). Use output P1 when operating in single-bridge configuration.
      | The modulating signals can be applied at Input 1 (Ust)
      | and the synchronization signal at input 2 (wt).
      |
      | Use 'Look_under mask' to get a description of the pulse pattern.
      mask init:
      | powericon('psbcbtransfo',gcb,'Discrete 3-phase PWM Generator');
      | if ModulatorType==1
      |     nPulses=6;
      |     SelectorElements=[1:1:12];
      | else
      |     nPulses=12;
      |  SelectorElements=[1:1:24];
      | end
      | if (ModulatingSignals==1 & ModulatorMode==2),
      |       CmdModulatingSignals=2;
      | else
      |       CmdModulatingSignals=1;
      | end
      mask StyleString: popup(2-level|3-level),popup(Synchronized|Un-synchronized),edit,edit,checkbox,edit,edit,edit,edit
      mask CallbackString: |powericon('psbcbtransfo',gcb,'Discrete 3-phase PWM Generator',2)|||powericon('psbcbtransfo',gcb,'Discrete 3-phase PWM Generator',5)||||
  Discrete Gamma Measurement : Subsystem  AncestorBlock=|  mask(Discrete Gamma Measurement (6-pulse converter)){transfo_type=Yg / Y, f0=60, Ith_min=0.001, Ts=50e-6}
      | powerlib_extras/Discrete 
      | Control Blocks/Discrete Gamma
      | Measurement
      mask prompts: transfo_type "Transformer connection:"; f0 "Base frequency (Hz):"; Ith_min "Current threshold for thyristor zero-current detection (pu or A):"; Ts "Sample time (s):"
      mask help:
      | This block measures the extinction angle Gamma for each of the 6 thyristors of a 6-pulse thyristor converter.
      |
      | Gamma is the time expressed in degrees from the thyristor current extinction to the time when the thyristor commutation voltage Vak becomes positive. The system frequency (input 3) is used to convert time values in electrical degrees. The current extinction time is determined from the "Current threshold" parameter (recommended value 0.1% of nominal current).
      | The 6 Gamma angles are determined using the 6 thyristor currents (input 1) and the 6 commutation voltages derived from the three phase-to-ground AC voltages measured at the primary of the converter transformer (input 2). The secondary winding connection of the converter transformer  (Y or Delta) is selectable from the "Transformer connection" parameter.
      |
      | The minimum value and the mean value of the 6 Gamma angles are sent respectively to output 1and output 2. Output 3 returns the 6 commutation voltages used in the determination of Gamma, assuming a 1:1 converter transformer ratio.
      mask StyleString: popup(Yg / Y|Yg / D1(lag)|Yg / D11(lead)),edit,edit,edit
      mask Display: disp('\n\n\n')
  Discrete HVDC Controller : Subsystem  mask(Discrete HVDC Controller){Mode=Rectifier (Current), XPILim=[166, 5], XLin=[160, 120], XKPI_I=[45, 4500, 90], Id_marg=0.1, XKPI_V=[35, 2250,  90], Vd_marg=0.05, XKPI_G=[1, 20,  90 ], G_marg=1, T_I=0.3e-3, XT_V=[15,  0.707], Xvdcol=[0.6, 0.18, 0.30, 0.1, 0.080], alpha_const=off, Xalpha_fix=[166, inf, -inf], dt=50e-6}
      mask prompts: Mode "Control Mode :"; XPILim "{Alpha Limits}  [alpha max (deg), alpha min (deg) ]"; XLin "Kp Lin. Angle Limits (alpha or beta) : [Max  (deg), Min  (deg) ]"; XKPI_I "{Current Regulator}   [Kp (deg/pu) , Ki (deg/pu/s), AlphaInit (deg) ]"; Id_marg "Current Margin (pu) :"; XKPI_V "{Voltage Regulator}   [Kp (deg/pu) , Ki (deg/pu/s),  AlphaInit (deg) ]"; Vd_marg "Voltage Margin (pu):"; XKPI_G "{Gamma Regulator} [Kp, Ki (s), AlphaInit (deg)]"; G_marg "Gamma Margin (deg):"; T_I "{Id Meas. Filter H(s)=1/(1+Ts)} T(s):"; XT_V "{Vd Meas. Low-Pass 2nd Order Filter}  [fo,  Zeta ]"; Xvdcol "{VDCOL}  [ VdThresh.(pu),VdMin(pu),IdMin(pu),IdMinAbs(pu),Tup(s) ]"; alpha_const "Constant alpha mode"; Xalpha_fix "{Ct.  or Forced alpha)}  [Alpha (deg), + Rate limit, - Rate limit (deg/s)]"; dt "Sample Time (s):"
      mask help:
      | This block contains the regulators and functions to control the firing angle alpha of a HVDC rectifier or inverter.
      |  See the 'HVDC Transmission System' case study of the User's Manual for description of the block functionality.
      mask init:
      | % Max_lin = max(180-Xlin)  Min_lin = min(180-Xlin)
      | 
      | alpha_max = XPILim(1); alpha_min = XPILim(2);
      | alpha_fix = Xalpha_fix(1); PRate_fix = Xalpha_fix(2);NRate_fix = Xalpha_fix(3);
      | Kp_I = XKPI_I(1); Ki_I = XKPI_I(2); ICi_I = XKPI_I(3);
      | Kp_V = XKPI_V(1); Ki_V = XKPI_V(2); ICi_V = XKPI_V(3);
      | Kp_G = XKPI_G(1); Ki_G = XKPI_G(2); ICi_G = XKPI_G(3);
      | f0_V = XT_V(1); Z_V = XT_V(2);
      | 
      | Inverter = Mode > 1;
      | 
      | if (Mode == 1) 
      | 	Id_marg = 0.0;
      | 	Max_lin = 60; Min_lin = 20;
      | else
      | 	Max_lin = 160; Min_lin = 120;
      | end;
      | 
      | 
      | Vd_seuil = Xvdcol(1); Vd_min=Xvdcol(2);Id_min=Xvdcol(3);Id_min_abs=Xvdcol(4);Tup=Xvdcol(5);
      | if strcmp(alpha_const,'on'), test_alpha = true; else, test_alpha = false; end
      mask StyleString: popup(Rectifier (Current)|Inverter (Current + Voltage + Gamma)|Inverter (Current + Voltage)|Inverter (Current + Gamma)),edit,edit,edit,edit,edit,edit,edit,edit,edit,edit,edit,checkbox,edit,edit
      mask CallbackString:
      | mode=get_param(gcb,'Mode');
      | 
      | cb=get_param(gcb,'MaskVisibilities');
      | 
      | if strcmp(mode,'Rectifier (Current)')
      | 	cb{10}='on';
      |     cb{11} = 'off';
      | 
      | 	 cb{3}='off';
      | 	 cb{5}='off';cb{6}='off';cb{7}='off';cb{8}='off';cb{9}='off';
      |     set_param(gcb,'MaskVisibilities',cb);
      | elseif (strcmp(mode,'Inverter (Current + Voltage + Gamma)'))
      | 	 cb{3}='off';
      | 	 cb{5}='on';cb{6}='on';cb{7}='on';cb{8}='on';cb{9}='on';cb{11} = 'on';
      | 	 set_param(gcb,'MaskVisibilities',cb);
      | elseif (strcmp(mode,'Inverter (Current + Voltage)'))
      | 	 cb{3}='off';
      | 	 cb{5}='on';cb{6}='on';cb{7}='on';cb{8}='off';cb{9}='off'; cb{11} = 'on';
      |      set_param(gcb,'MaskVisibilities',cb);
      | else
      | 	 cb{3}='off';
      | 	 cb{5}='on';cb{6}='off';cb{7}='off';cb{8}='on';cb{9}='on'; cb{11} = 'on';
      | 	 set_param(gcb,'MaskVisibilities',cb);
      | end||||||||||||||
  Discrete SV PWM Generator : Subsystem  mask(Discrete SV PWM Generator){InputType=Magnitude-Angle (rad), SwitchingPattern=Pattern #1, Fc=2000, ParUref=[0.8 -30 50], Ts=2e-6}
      mask prompts: InputType "Data type of input reference vector (U*):"; SwitchingPattern "Switching pattern:"; Fc "Chopping frequency (Hz):"; ParUref "Output voltage: [ Mag(0<m<1) Phase(deg.)  Freq(Hz) ]"; Ts "Sample time:"
      mask help:
      | This block generates pulses for a three-phase basic two-level voltage-sourced converter (VSC) consisting of three half-bridge switching devices (FETs, GTOs or IGBTs).
      | The block utilizes the space vector pulse width modulation (SV PWM) technique to generate firing pulses to the 6 switching devices of the converter. Two switching patterns can be selected.
      | The modulation index m (magnitude of the reference vector U) must be a value between 0 and 1.
      | The line-to-line rms voltage generated by a VSC controlled by this block will be: Vout= m * Vdc / sqrt(2).
      mask init:
      | powericon('DSVPWMGeneratorCback',gcb);
      | m=ParUref(1);
      | Pha=ParUref(2);
      | Freq=ParUref(3);
      mask StyleString: popup(Magnitude-Angle (rad)|alpha-beta components|Internally generated),popup(Pattern #1|Pattern #2),edit,edit,edit
      mask CallbackString: powericon('DSVPWMGeneratorCback',gcb);||||
  Discrete Synchronized 12-Pulse Generator : Subsystem  mask(Discrete synchronized 12-pulse generator){pwidth=10, Double_Pulse=on, Ts=Ts}
      mask prompts: pwidth "Pulse width (degrees) :"; Double_Pulse "Double pulsing"; Ts "Sample time:"
      mask help:
      | Use his block  to fire the 12 thyristors of a 12-pulse converter.
      | Outputs 1 and 2 are two vectors of 6 pulses (0-1) to be sent to the two 6-pulse half bridges connected respectively to the Wye(Y) and Delta (D) connected windings of the YYD (Delta lagging) converter transformer. Pulses are individually synchronized on the 6 commutation voltages and generated alpha degrees after the increasing zero-crossings of the commutation voltages. The D pulses are lagging the Y pulses by  30 degrees.
      |
      | Input 1 is  the alpha firing signal (degrees).
      | Inputs 2, 3 and 4 are the three phase-ground synchronization voltages  measured at the  primary side of the converter transformer.
      | Input 5: Frequency of the synchronization voltages (use a constant or the Freq PLL output)
      | Input 6 allows  blocking of the pulses when the applied signal is non zero.
      |
      | When the 'Douple pulsing' option is checked, two pulses are sent to each thyristor: a 1st pulse when the aplha angle is reached, then a 2nd pulse 60 degrees later, when the next thyristor is fired.
      mask Display: plot(0,0,100,100,[80 62 62 47 47 30],[40 40 60 60 40 40]-5)
  Discrete Synchronized 6-Pulse Generator : Subsystem  mask(Discrete Synchronized 6-pulse generator){pwidth=10, Double_Pulse=on, Ts=Ts}
      mask prompts: pwidth "Pulse width (degrees) :"; Double_Pulse "Double pulsing"; Ts "Time step (s) :"
      mask help:
      | Use this block to fire the 6 thyristors of a 6-pulse converter.
      |
      | The output is a vector of 6 pulses (0-1) individually synchronized on the 6 commutation voltages. Pulses are generated alpha degrees after the increasing zero-crossings of the commutation voltages.
      |
      | Input 1 is  the alpha firing signal (degrees).
      | Inputs 2, 3 and 4 are the synchronization voltages AB BC CA which should be in phase with the 3 phase-phase voltages at the converter terminals.
      | Input 5: Frequency of the synchronization voltages (use a constant or the Freq PLL output)
      | Input 6 allows  blocking of the pulses when the applied signal is non zero.
      |
      | When the 'Douple pulsing' option is checked, two pulses are sent to each thyristor: a 1st pulse when the aplha angle is reached, then a 2nd pulse 60 degrees later, when the next thyristor is fired.
      mask Display: plot(0,0,100,100,[80 62 62 47 47 30],[40 40 60 60 40 40]-5)
  Discrete Variable Transport Delay : Subsystem  mask(Discrete variable transport delay){MaxDelay=1/40, InitialValue=0, Ts=50e-6}
      mask prompts: MaxDelay "Maximum delay (s):"; InitialValue "Initial input:"; Ts "Sample time:"
      mask help:
      | Apply a delay to the first input (In) signal.
      | The second input (D) specifies the delay time.
  Timer : powerlib_extras/Control  Blocks/Timer  t="[ 0  1  3  3.5  ]"  e="[1  -1  2.5  0   ]"
